simulink library "UAV_Control"  (R2018a)
settings: Solver=ode45  StartTime=0.0  StopTime=10.0  RelTol=1e-3  EnableMultiTasking=on
undefined symbols (not defined in the file or in its folder): alpha, dc_M_z, delta, Epsilon, g, Gamma, gamma_0, gamma_d_z, h, k, K, Ky, L, magnitude, mu1, mu2, nu, omega0, omega1, omega2, Phi0, Psi0, Rate, Rho_L, Rho_M, RPM_per, Sat, t0, t1, Tau, theta, theta0, Theta0, theta_0, theta_dot_M, theta_Max, theta_Min, Thrust_per, Tm, v, V0, X0, Xmax, Xmin, zeta1, zeta2, Zg
libraries: simulink x12, $bdroot x7
(part 1 of 2)
settings Model: Creator=ahmad  LastModifiedBy=Ahmad
settings DataIOCC: LimitDataPoints=on
settings OptimizationCC: LifeSpan=inf
settings DebuggingCC: AllowSymbolicDim=off  SFUnexpectedBacktrackingDiag=warning  SFNoUnconditionalDefaultTransitionDiag=warning  SFExecutionAtInitializationDiag=none
settings CodeAppCC: StateflowObjectComments=on
settings GRTTargetCC: TargetLangStandard=C89/C90 (ANSI)  GeneratePreprocessorConditionals=Disable all
settings ConfigComp: CovMetricSettings=dw  CovHtmlReporting=on  CovSaveCumulativeToWorkspaceVar=on  CovSaveSingleToWorkspaceVar=on  CovExternalEMLEnable=off

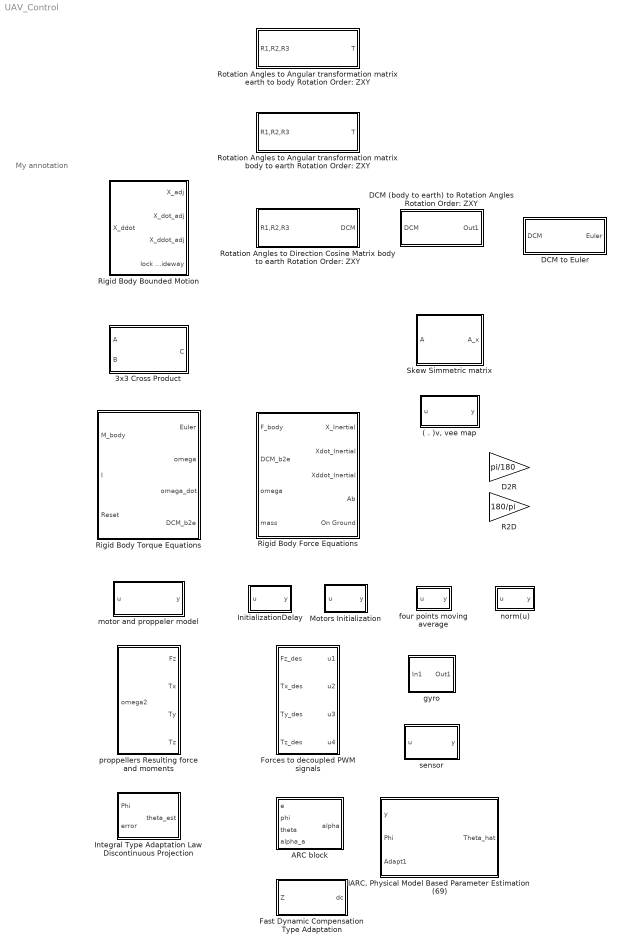
== system UAV_Control ==
  note: My annotation
  "( . )v, vee map" : Subsystem
  3x3 Cross Product : Subsystem  mask(3x3 Cross prduct){}
      mask Display:
      | port_label('input',1,'A','texmode','on')
      | port_label('input',2,'B','texmode','on')
      | port_label('output',1,'C','texmode','on')
  ARC block : Subsystem  mask(ARCBlock){k=k, theta_max=theta_Max, theta_min=theta_Min, epsilon=Epsilon, delta=delta}
      mask prompts: k "Linear Robuts gain:"; theta_max "Maximum parameters vector value:"; theta_min "Minimum parameters vector value:"; epsilon "Error bound Coefficient:"; delta "Uncertain Nonlinearities Bound:"
      mask help: Computes the ARC control part including: model compensation, stabalizing feedback, nonlinear robust feedback.
      mask Help:
      | h^2=(theta_max-theta_min)^2*phi^2+delta^2
      | alpha= alpha_a-( k + h^2/(4epsilon) )e/theta
      mask Display:
      | port_label('input',1,'e','texmode','on')
      | port_label('input',2,'\phi','texmode','on')
      | port_label('input',3,'\theta','texmode','on')
      | port_label('input',4,'\alpha_a','texmode','on')
      | port_label('output',1,'\alpha','texmode','on')
  "D2R " : Gain  Gain=pi/180  SaturateOnIntegerOverflow=on  OutDataTypeStr=Inherit: Same as input  ParamDataTypeStr=Inherit: Same as input
  DCM (body to earth) to Rotation Angles Rotation Order: ZXY : Subsystem  mask(DCM2Ang){}
      mask help: Get Euler angles from DCM in ZXY format.
      mask Help: Get Euler angles from DCM in ZXY format.
      mask Display:
      | port_label('input',1,'DCM_{be}','texmode','on')
      | port_label('output',1,'[R_1,R_2,R_3]','texmode','on')
  DCM to Euler : Subsystem
  Fast Dynamic Compensation Type Adaptation : Subsystem  mask{dc_M=dc_M_z, gamma_d=gamma_d_z}
      mask prompts: dc_M "Bound for the lumped model compensation errors"; gamma_d "Adaptation gain:"
      mask Help:
      | d ̂  ̇_c=Proj(γ_d z)=0             if      |d ̂_c |=d_cM  and d ̂_c z>0
      |                                 γ_d z      else
      | With γ_d>0 and |d ̂_c (0)|≤d_cM
      mask Display:
      | port_label('input',1,'e','texmode','on')
      | port_label('output',1,'d_c','texmode','on')
  Forces to decoupled PWM signals : Subsystem  mask(Forces2PWMSignals){K=K, Ky=Ky, L=L}
      mask prompts: K "Proppeler Force Coefficient:"; Ky "Proppeler Torque Coefficient:"; L "Arm Length:"
      mask help: Convertes the Quadcopter desired forces and moments to equivalent PWM signal.
      mask Help:
      | Convertes the Quadcopter desired forces and moments to equivalent PWM signal for a specific motors configuration.
      | 
      | Motors indices and rotation direction:
      | 1: back (CW)
      | 2: front (CW)
      | 3: left (CCW)
      | 4: righ (CCW)
      | 
      | parameters:
      | K: Proppeler Force Coefficient (N/(rad/s)^2)
      | Ky: Proppeler Torque Coefficient (N.m/(rad/s)^2)
      | L: Arm Length (m)
      | 
      | Inputs:
      | Fn=F/(4K)
      | Txn=Tx/(2LK)
      | Tyn=Ty/(2LK)
      | Tzn=Tz/(4Ky)
      | 
      | Outputs:
      | u1 =sqrt( Fn + Tyn + Tzn)
      | u2 = sqrt(Fn - Tyn + Tzn)
      | u3 = sqrt(Fn + Txn - Tzn)
      | u4 = sqrt(Fn - Txn - Tzn)
      | 
      | The PWM Duty cylce (ui) is limeted between 0 and 1.
      mask Display:
      | port_label('input',1,'F_{z,des}','texmode','on')
      | port_label('input',2,'\tau_{x,des}','texmode','on')
      | port_label('input',3,'\tau_{y,des}','texmode','on')
      | port_label('input',4,'\tau_{z,des}','texmode','on')
      | port_label('output',1,'u1','texmode','on')
      | port_label('output',2,'u2','texmode','on')
      | port_label('output',3,'u3','texmode','on')
      | port_label('output',4,'u4','texmode','on')
  "IARC, Physical Model Based Parameter Estimation (69)" : Subsystem  mask(Physical Model Based Parameter Estimation){mu1=mu1, mu2=mu2, alpha=alpha, nu=nu, gamma0=gamma_0, Rho_M=Rho_M, Rho_L=Rho_L, v=v, theta_0=theta_0, theta_max=theta_Max, theta_min=theta_Min, Theta_dot_M=theta_dot_M, Tau=Tau, t0=t0, Norm_ON=on}
      mask prompts: mu1 "forgetting factor, mu1:"; mu2 "RLS parameter, mu2:"; alpha "forgetting factor, alpha:"; nu "normalizing factor, nu:"; gamma0 "Initial adaptation gain:"; Rho_M "Upper bound for the adaptation gain:"; Rho_L "Lower bound for the adaptation gain:"; v "Eigenvector of Gamma_max:"; Theta_dot_M "Theta dot max:"; Tau "Filter time constant:"; t0 "Initialization Delay:"; Norm_ON "Use Normalized formula"
      mask Help:
      | Filtered system dynamics:
      | H_f (s)  is any stable LTI filter transfer function
      | x_f=H_f [x]
      | φ_f=H_f [φ(x)]
      | u_f=H_f [u]
      | 
      | y_p=x ̇_f−u_f
      | y ̂_p=φ_f^T θ ̂
      | Prediction error:
      | ϵ=y_p−y ̂_p
      | 
      | recursive estimation algorithms, the generalized parameter estimation algorithm (PAA) with covariance limiting:
      | 
      | θ ̂  ̇(t)=Γ(t) φ_f (t)ϵ(t)
      | D_Γ=μ_1 (t)Γ(t)−μ_2 (t)Γ(t) φ_f (t) φ_f (t)^T Γ(t)
      | Γ ̇(t)=D_Γ, if λ_M (Γ(t))<ρ_M  or v_M^T D_Γ v_M<0 )
      |          0        else
      | 
      | μ_1  and μ_2  are two non-negative functions
      | ρ_M  is a preset upper bound for the covariance matrix Γ(t)
      | μ_1  represents the forgetting factor (μ_1=0 for not forgetting)
      | μ_2: 1 stands for the standard least squares type estimation algorithm
      |        0 stands for  the gradient type estimation algorithm
      |        range: 0≤μ_2<2
      | Initialization of the covariance matrix: Γ(0)<ρ_M I_p
      | 
      | IARC designs completely separate the parameter estimation law design from the underlying robust control law to give better parameter estimates than possible with DARC designs. In addition, explicit on-line signal excitation level monitoring can be employed to significantly improve the accuracy of  parameter estimates.
      | 
      | Normalized Method:
      | θ ̂  ̇(t)=(Γ(t) φ_f (t)ϵ(t))/(1+νφ_f^T Γφ_f )
      | D_Γ=αΓ(t)−(Γ(t) φ_f (t) φ_f (t)^T Γ(t))/(1+νφ_f^T Γφ_f )
      | Γ ̇(t)=D_Γ, if λ_M (Γ(t))<ρ_M  or v_M^T D_Γ v_M<0
      |           0       else
      mask Display:
      | port_label('input',1,'y','texmode','on')
      | port_label('input',2,'\phi','texmode','on')
      | port_label('input',3,'Adapt','texmode','on')
      | 
      | port_label('output',1,'\theta_{hat}','texmode','on')
  InitializationDelay : Subsystem  mask(InitializationDelay){t0=t0}
      mask prompts: t0 "Initialization delay:"
      mask help: Applays a delay before passing the first signal.
      mask Help: Applays a delay (t0) before passing the first signal
      mask Display:
      | port_label('input',1,'u','texmode','on')
      | port_label('output',1,'y','texmode','on')
  Integral Type Adaptation Law Discontinuous Projection : Subsystem  mask(IntegralTypeAdaptationLaw){theta=theta, theta0=theta0, theta_max=theta_Max, theta_min=theta_Min, gamma=Gamma, t0=t0, Adaptation_ON=on}
      mask prompts: theta "Actual value of theta:"; theta0 "Initial value of theta:"; theta_max "Maximum value of theta:"; theta_min "Minimum value of theta:"; gamma "Adaptation Rate:"; t0 "Initialization Delay:"; Adaptation_ON "Activate adaptation:"
      mask help: Applies an Integral-type adaptation law with discontinuous projection on the parameter theta.
      mask Help:
      | Applies an Integral-type adaptation law with discontinuous projection on the parameter theta.
      | 
      | theta_est_dot=Gamma*Phi*e
      | theta=proj( int(theta_estdot) )
      | 
      | theta_min < theta_est <  theta_max
      | 
      | Parameters:
      | 
      | Gamma: nxn diagonal matrix, adaptaion rate.
      | theta_min: nx1 vector, minimum value of the estimated vector.
      | theta_max: nx1 vector, maximum value of the estimated vector.
      | theta0: nx1 vector, initial value of the estimated vector.
      | theta: nx1 vector, actual value of the estimated vector.
      | Adaptation_On: controls the use of the adaptation law (1: active, 0: inactive)
      | 
      | Inputs:
      | Phi: regressor vector, theta0, nx1.
      | e: state error, scalar.
      | 
      | Outputs:
      | theta_est: estimated value of the parameters vector.
      mask Display:
      | port_label('input',1,'\phi','texmode','on')
      | port_label('input',2,'e','texmode','on')
      | port_label('output',1,'\theta_{hat}','texmode','on')
  "Motors Initialization " : Subsystem  mask(MotorsInitialization){t0=t0, t1=t1, Sat=Sat, Parameter4=Rate}
      mask prompts: t0 "Initialization delay:"; t1 "Input pass time:"; Sat "Signal saturation during initialization:"; Parameter4 "Signal rate during initialization:"
      mask help: Delays the pass out of the input while passing a warmup rizing signal.
      mask Display:
      | port_label('input',1,'u','texmode','on')
      | port_label('output',1,'y','texmode','on')
  "R2D " : Gain  Gain=180/pi  SaturateOnIntegerOverflow=on  OutDataTypeStr=Inherit: Same as input  ParamDataTypeStr=Inherit: Same as input
  Rigid Body Force Equations : Subsystem  mask(Rigid body force equations){g=g, h0=Zg, X0=X0, X_min=Xmin, X_max=Xmax, V0=V0}
      mask prompts: g "Gravity:"; h0 "Ground height:"; X0 "Initial Position:"; X_min "Position Lower Bound:"; X_max "Position Upper Bound:"; V0 "Initial Velocity:"
      mask help: Determines the translational motion of a 6DOF rigid body.
      mask Help:
      | a_b= Fb/m-omega x V_b
      | 
      | 
      | 
      | Fb=R_eb*[0 0 -mg]+[0 0 Fz]+R_eb*Fd_e
      | 
      | where Fz is the thrust force (in body z direction)
      | and Fd_e is a force disturbace in the earth frame.
      | 
      | a_e = R_be*a_b
      mask Display:
      | port_label('input',1,'F_b (N)','texmode','on')
      | port_label('input',2,'DCM_{b2e}','texmode','on')
      | port_label('input',3,'\omega (rad/s)','texmode','on')
      | port_label('input',4,'m (kg)','texmode','on')
      | 
      | port_label('output',1,'X_e (m)','texmode','on')
      | port_label('output',2,'V_e (m/s)','texmode','on')
      | port_label('output',3,'a_e (m/s^2)','texmode','on')
      | port_label('output',4,'a_b (m/s^2)','texmode','on')
      | port_label('output',5,'On Ground','texmode','on')
  "Rigid Body Torque Equations " : Subsystem  mask(Rotational motion of rigid body){Euler0=[Phi0 Theta0 Psi0], omega0=omega0}
      mask prompts: Euler0 "Initial euler angles:"; omega0 "Initial angular velocites:"
      mask help: Determines the rotational motion of a 6DOF rigid body.
      mask Help:
      | alpha=Mb/I - omega x omega
      | omega=alpha_dot
      | Euler=omega_dot
      mask Display:
      | port_label('input',1,'M_b (N.m)','texmode','on')
      | port_label('input',2,'I (kg/m^2)','texmode','on')
      | port_label('input',3,'Reset','texmode','on')
      | 
      | port_label('output',1,'\phi,\theta,\psi (rad)','texmode','on')
      | port_label('output',2,'\omega (rad/s)','texmode','on')
      | port_label('output',3,'\alpha (rad/s^2)','texmode','on')
      | port_label('output',4,'DCM_{b2e}','texmode','on')
  Rigid Body Bounded Motion : Subsystem  mask{Parameter1=Zg, Parameter2=X0, Parameter3=V0, Parameter4=Xmin, Parameter5=Xmax}
      mask prompts: Parameter1 "Ground level:"; Parameter2 "Initial Possition:"; Parameter3 "Initial Velocity:"; Parameter4 "Position Lower Bound:"; Parameter5 "Position Upper Bound:"
      mask help: Bounds the motion of a rigid body in space: [Xmin Xmax]
      mask Help:
      | Bounds the motion of a rigid body in space.
      | 
      | Dialog box parameters:
      | Zg: A scalar value for ground height (m).
      | X0 (x,y,z): tree-element vector, initial position of the body (m).
      | V0(vx,vy,vz): tree-element vector, for the initial velocity of the body (m/s).
      | Xmin: tree-element vector for the position lower bound (m).
      | Xmax: tree-element vector for the position upper bound (m).
      | 
      | Input:
      | First: Contains the acceleration of the body resolved into the earth coordinate frame, (A, m/s).
      | 
      | Outputs:
      | First: Contains the bounded position of the body resolved into the earth coordinate frame, tree-element vector, (X, m).
      | Second: Contains the bounded velocitiy of the body resolved into the earth coordinate frame, tree-element vector, (Vadj, m/s).
      | Third: Contains the bounded acceleration of the body resolved into the earth coordinate frame, tree-element vector, (Aadj, m/s2).
      mask Display:
      | port_label('input',1,'A','texmode','on');
      | port_label('output',1,'X_{b}','texmode','on');
      | port_label('output',2,'V_{adj}','texmode','on');
      | port_label('output',3,'A_{adj}','texmode','on');
      | port_label('output',4,'On ground','texmode','on');
  Rotation Angles to Angular transformation matrix body to earth Rotation Order: ZXY : Subsystem  mask(Ang2T){}
      mask help: Determine the 3-by-3 Angular transformation matrix (T) from a given set of rotation angles (ZXY).
      mask Help:
      | Generate the Angular Transformation matrix (T) from the Euler angles. Order of transformation. body to earth.
      | ZYX
      | 
      | T_B2E = [         cos(theta)             0          -sin(theta)
      |                  -sin(theta)*tan(phi)      1    -cos(theta)*tan(phi)
      |                    sin(theta)/cos(phi)     0     cos(theta)/cos(phi) ]
      mask Display:
      | port_label('input',1,'[R_1,R_2,R_3]','texmode','on')
      | port_label('output',1,'T_{eb}','texmode','on')
  Rotation Angles to Angular transformation matrix earth to body Rotation Order: ZXY : Subsystem  mask(Ang2T){}
      mask help: Determine the 3-by-3 Angular transformation matrix (T) from a given set of rotation angles (ZXY).
      mask Help:
      | Generate the Angular transformation matrix  (T) from the Euler angles. Order of transformation.
      | ZXY
      | 
      | T_B2E = [         cos(theta)             0          -sin(theta)*cos(phi)
      |                                0                       1                    sin(phi)
      |                          sin(theta)              0            cos(theta)*cos(phi) ]
      mask Display:
      | port_label('input',1,'[R_1,R_2,R_3]','texmode','on')
      | port_label('output',1,'T_{eb}','texmode','on')
  Rotation Angles to Direction Cosine Matrix body to earth Rotation Order: ZXY : Subsystem  mask(Ang2DCM){}
      mask help: Determine the 3-by-3 direction cosine matrix (DCM) from a given set of rotation angles.
      mask Help:
      | Generate the Direction Cosine Matrix (DCM) from the Euler angles. Order of transformation: ZXY.
      | ZYX >> phi theta psi
      | 
      | DCM_B2E=[cos(theta)cos(psi), sin(phi)sin(theta)cos(psi)-cos(phi)sin(psi), cos(phi)sin(theta)cos(psi)+sin(phi)sin(psi)
      |                       cos(theta)sin(psi), sin(phi)sin(theta)sin(psi)+cos(phi)cos(psi), cos(phi)sin(theta)sin(psi)-sin(phi)cos(psi)
      |                             -sin(theta)      ,                 sin(phi)cos(theta)                          ,                           cos(phi)cos(theta)               ]
      | 'texmode','on'
      mask Display:
      | port_label('input',1,'[R_1,R_2,R_3]','texmode','on')
      | port_label('output',1,'DCM_{eb}','texmode','on')
  Skew Simmetric matrix : Subsystem
  four points moving average : Subsystem
  gyro : Subsystem
  motor and proppeler model : Subsystem  mask{CorrMode=off, Thrust=Thrust_per, RPM=RPM_per, TimeConstant=Tm}
      mask prompts: CorrMode "Correction mode"; Thrust "Thrust percentage data:"; RPM "RPM percentage data:"; TimeConstant "Motor time constant:"
      mask init:
      | if CorrMode
      |     c=1;
      | else
      |     c=0;
      | end
      mask Display:
      | port_label('input',1,'Duty cycle','texmode','on')
      | port_label('output',1,'\omega^2','texmode','on')
  norm(u) : Subsystem
  proppellers Resulting force and moments : Subsystem  mask(QuadcopterMotorsResultingForces&Moments){K=K, Ky=Ky, L=L}
      mask prompts: K "Proppeler Force Coefficient:"; Ky "Proppeler Torque Coefficient:"; L "Arm Length:"
      mask help: Calculates the resulting forces & moments of the quadcopter motors.
      mask Help:
      | Calculates the resulting forces & moments of the quadcopter motors given the motors speed.
      | 
      | parameters:
      | K: Proppeler Force Coefficient (N/(rad/s)^2)
      | Ky: Proppeler Torque Coefficient (N.m/(rad/s)^2)
      | L: Arm Length (m)
      | 
      | Fz=K*(omega1^2+omega2^2+omega3^2+omega4^2)
      | Tx=K*L*(omega3^2-omega4^2)
      | Ty=K*L*(omega1^2-omega2^2)
      | Tz=Ky*(omega1^2+omega2^2-omega3^2-omega4^2)
      | 
      | Input:
      | omega^2: a four elements vector contaning the squared velocity of each of the four motors.
      | 
      | Outputs:
      | all the outputs are in body frame.
      | Fz: Total force in the Z direction.
      | Tx: Moment about the body X-axis.
      | Ty: Moment about the body Y-axis.
      | Tz: Moment about the body Z-axis.
      mask Display:
      | port_label('input',1,'\omega^2','texmode','on')
      | port_label('output',1,'F_z','texmode','on')
      | port_label('output',2,'\tau_x','texmode','on')
      | port_label('output',3,'\tau_y','texmode','on')
      | port_label('output',4,'\tau_z','texmode','on')
  sensor : Subsystem

== system UAV_Control/( . )v, vee map ==
  u : Inport
  12 (D_psi) : Selector  NumberOfDimensions=2  InputPortWidth=3  IndexOptions=Index vector (dialog),Index vector (dialog)  Indices=1,2  OutputSizes=1,1
  23 (D_phi) : Selector  NumberOfDimensions=2  InputPortWidth=3  IndexOptions=Index vector (dialog),Index vector (dialog)  Indices=2,3  OutputSizes=1,1
  31 (D_theta) : Selector  NumberOfDimensions=2  InputPortWidth=3  IndexOptions=Index vector (dialog),Index vector (dialog)  Indices=3,1  OutputSizes=1,1
  Mux : Mux  Inputs=3
  y : Outport
  wires:
  12 (D_psi)/1 -> Mux/3
  31 (D_theta)/1 -> Mux/2
  23 (D_phi)/1 -> Mux/1
  u/1 -> 31 (D_theta)/1, 23 (D_phi)/1, 12 (D_psi)/1
  Mux/1 -> y/1

== system UAV_Control/3x3 Cross Product ==
  A : Inport
  B : Inport  Port=2
  "A " : InportShadow
  "B " : InportShadow  Port=2
  Subsystem : Subsystem
  Subsystem1 : Subsystem
  Sum : Sum  Inputs=+|-  SaturateOnIntegerOverflow=on  InputSameDT=on  OutDataTypeStr=Inherit: Same as first input
  C : Outport
  wires:
  Subsystem1/1(Out1) -> Sum/2
  Subsystem/1(Out1) -> Sum/1
  A/1 -> Subsystem/1(A)
  B/1 -> Subsystem/2(B)
  Sum/1 -> C/1
  "A "/1 -> Subsystem1/1(A)
  "B "/1 -> Subsystem1/2(B)

== system UAV_Control/ARC block ==
  e : Inport
  phi : Inport  Port=2
  theta : Inport  Port=3
  alpha_a : Inport  Port=4
  1 : Scope
  Add : Sum  Inputs=--+
  Mux1 : Mux
  alpha_S1 : Gain  Gain=k
  e/theta : Product  Inputs=*/
  h^2 : Subsystem
      mask Display:
      | port_label('input',1,'e/\theta','texmode','on')
      | port_label('input',2,'\phi','texmode','on')
      | 
      | port_label('output',1,'\alpha_{s2}','texmode','on')
  alpha : Outport
  wires:
  e/theta/1 -> alpha_S1/1, h^2/1(e)
  alpha_a/1 -> Mux1/3, Add/3
  Mux1/1 -> 1/1
  Add/1 -> Mux1/4, alpha/1
  alpha_S1/1 -> Mux1/1, Add/1
  h^2/1("alpha_s2 ") -> Mux1/2, Add/2
  e/1 -> e/theta/1
  theta/1 -> e/theta/2
  phi/1 -> h^2/2(phi)

== system UAV_Control/DCM (body to earth) to Rotation Angles Rotation Order: ZXY ==
  DCM : Inport  Unit=1
  "AxisRotDefault " : Subsystem  TreatAsAtomicUnit=on
  "AxisRotZeroR3 " : Subsystem  TreatAsAtomicUnit=on
  "Get DCM Values " : Subsystem
  If : If  IfExpression=(u1>=1)|(u1<=-1)
  Merge : Merge
  Selector4 : Selector  InputPortWidth=7  IndexOptions=Index vector (dialog)  Indices=3  OutputSizes=1
  Out1 : Outport  Unit=rad
  wires:
  "AxisRotZeroR3 "/1(Out1) -> Merge/1
  "AxisRotDefault "/1(Out1) -> Merge/2
  If/2 -> "AxisRotDefault "/Action
  Merge/1 -> Out1/1
  Selector4/1 -> If/1  "r21"
  "Get DCM Values "/1(Out1) -> "AxisRotZeroR3 "/1(In1), "AxisRotDefault "/1(In1), Selector4/1
  DCM/1 -> "Get DCM Values "/1(In1)
  If/1 -> "AxisRotZeroR3 "/Action

== system UAV_Control/DCM to Euler ==
  DCM : Inport
  12 : Selector  NumberOfDimensions=2  InputPortWidth=3  IndexOptions=Index vector (dialog),Index vector (dialog)  Indices=1,2  OutputSizes=1,1
  22 : Selector  NumberOfDimensions=2  InputPortWidth=3  IndexOptions=Index vector (dialog),Index vector (dialog)  Indices=2,2  OutputSizes=1,1
  31 : Selector  NumberOfDimensions=2  InputPortWidth=3  IndexOptions=Index vector (dialog),Index vector (dialog)  Indices=3,1  OutputSizes=1,1
  32 : Selector  NumberOfDimensions=2  InputPortWidth=3  IndexOptions=Index vector (dialog),Index vector (dialog)  Indices=3,2  OutputSizes=1,1
  33 : Selector  NumberOfDimensions=2  InputPortWidth=3  IndexOptions=Index vector (dialog),Index vector (dialog)  Indices=3,3  OutputSizes=1,1
  Mux : Mux  Inputs=3
  Mux1 : Mux  Inputs=3
  Mux2 : Mux  Inputs=3
  phi : Fcn  Expr=asin(u(1))
  psi : Fcn  Expr=atan2(-u(1)/cos(u(3)),u(2)/cos(u(3)))
  theta : Fcn  Expr=atan2(-u(1)/cos(u(3)),u(2)/cos(u(3)))
  Euler : Outport
  wires:
  psi/1 -> Mux2/3
  Mux1/1 -> psi/1
  Mux/1 -> theta/1
  33/1 -> Mux/2
  32/1 -> phi/1
  DCM/1 -> 12/1, 22/1, 33/1, 32/1, 31/1
  22/1 -> Mux1/2
  12/1 -> Mux1/1
  phi/1 -> Mux1/3, Mux2/1, Mux/3
  theta/1 -> Mux2/2
  31/1 -> Mux/1
  Mux2/1 -> Euler/1

== system UAV_Control/Fast Dynamic Compensation Type Adaptation ==
  Z : Inport
  Gain : Gain  Gain=gamma_d
  Integrator : Integrator  LimitOutput=on  UpperSaturationLimit=dc_M  LowerSaturationLimit=-dc_M
  dc : Outport
  wires:
  Integrator/1 -> dc/1
  Z/1 -> Gain/1
  Gain/1 -> Integrator/1

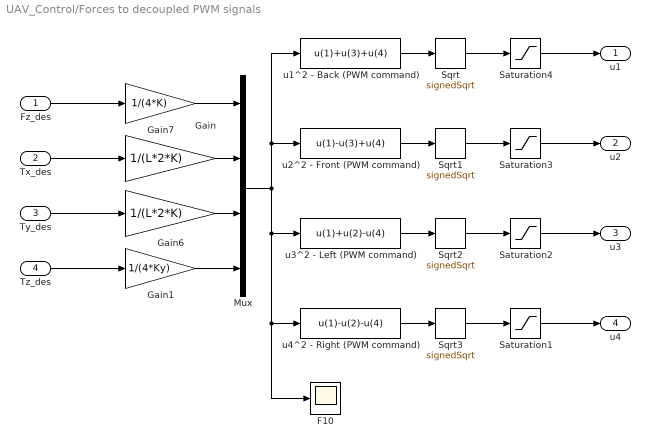
== system UAV_Control/Forces to decoupled PWM signals ==
  Fz_des : Inport
  Tx_des : Inport  Port=2
  Ty_des : Inport  Port=3
  Tz_des : Inport  Port=4
  F10 : Scope
  Gain : Gain  Gain=1/(L*2*K)
  Gain1 : Gain  Gain=1/(4*Ky)
  Gain6 : Gain  Gain=1/(L*2*K)
  Gain7 : Gain  Gain=1/(4*K)
  Mux : Mux
  Saturation{1..4} (4 alike) : Saturate  UpperLimit=1  LowerLimit=0
  Sqrt{,1..3} (4 alike) : Sqrt  Operator=signedSqrt  OutputSignalType=real  SaturateOnIntegerOverflow=on
  u1^2 - Back (PWM command) : Fcn  Expr=u(1)+u(3)+u(4)
  u2^2 - Front (PWM command) : Fcn  Expr=u(1)-u(3)+u(4)
  u3^2 - Left (PWM command) : Fcn  Expr=u(1)+u(2)-u(4)
  u4^2 - Right (PWM command) : Fcn  Expr=u(1)-u(2)-u(4)
  u1 : Outport
  u2 : Outport  Port=2
  u3 : Outport  Port=3
  u4 : Outport  Port=4
  wires:
  Sqrt1/1 -> Saturation3/1
  Sqrt2/1 -> Saturation2/1
  Sqrt3/1 -> Saturation1/1
  Sqrt/1 -> Saturation4/1
  u4^2 - Right (PWM command)/1 -> Sqrt3/1
  u3^2 - Left (PWM command)/1 -> Sqrt2/1
  u2^2 - Front (PWM command)/1 -> Sqrt1/1
  u1^2 - Back (PWM command)/1 -> Sqrt/1
  Saturation1/1 -> u4/1
  Saturation3/1 -> u2/1
  Saturation2/1 -> u3/1
  Saturation4/1 -> u1/1
  Gain7/1 -> Mux/1
  Gain1/1 -> Mux/4
  Gain6/1 -> Mux/3
  Gain/1 -> Mux/2
  Mux/1 -> u1^2 - Back (PWM command)/1, u2^2 - Front (PWM command)/1, u3^2 - Left (PWM command)/1, u4^2 - Right (PWM command)/1, F10/1
  Tz_des/1 -> Gain1/1
  Ty_des/1 -> Gain6/1
  Fz_des/1 -> Gain7/1
  Tx_des/1 -> Gain/1

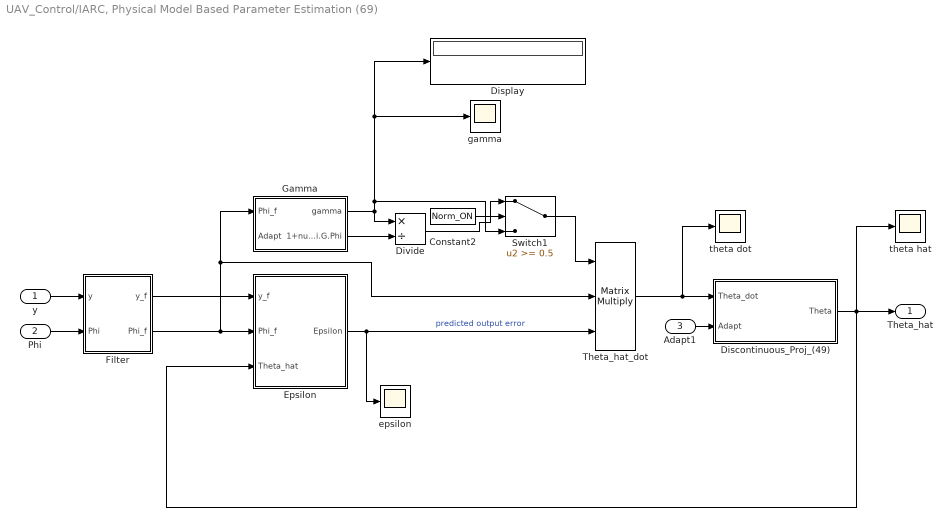
== system UAV_Control/IARC, Physical Model Based Parameter Estimation (69) ==
  y : Inport
  Phi : Inport  Port=2
  Adapt1 : Inport  Port=3
  Constant2 : Constant  Value=Norm_ON
  Discontinuous_Proj_(49) : Subsystem
  Display : Display
  Divide : Product  Inputs=*/
  Epsilon : Subsystem
  Filter : Subsystem
  Gamma : Subsystem
  Switch1 : Switch  Threshold=0.5
  Theta_hat_dot : Product  Inputs=3  Multiplication=Matrix(*)
  "epsilon  " : Scope
  gamma : Scope
  theta dot : Scope
  theta hat : Scope
  Theta_hat : Outport
  wires:
  Gamma/2(" 1+nu.Phi.G.Phi") -> Divide/2
  Divide/1 -> Switch1/1
  Switch1/1 -> Theta_hat_dot/1
  Gamma/1(" gamma") -> Divide/1, Switch1/3, gamma/1, Display/1
  Constant2/1 -> Switch1/2
  Theta_hat_dot/1 -> theta dot/1, Discontinuous_Proj_(49)/1(Theta_dot)
  y/1 -> Filter/1(y)
  Phi/1 -> Filter/2("Phi ")
  Filter/1(y_f) -> Epsilon/1(y_f)
  Discontinuous_Proj_(49)/1(Theta) -> theta hat/1, Theta_hat/1, Epsilon/3(Theta_hat)
  Epsilon/1(Epsilon) -> Theta_hat_dot/3, "epsilon  "/1  "predicted output error"
  Filter/2(Phi_f) -> Theta_hat_dot/2, Gamma/1(Phi_f), Epsilon/2(Phi_f)
  Adapt1/1 -> Discontinuous_Proj_(49)/2(Adapt)

== system UAV_Control/InitializationDelay ==
  u : Inport
  Clock : Clock
  Compare To Constant2 : simulink/Logic and Bit Operations/Compare To Constant  relop=>=  const=t0  OutDataTypeStr=boolean
  Data Type Conversion : DataTypeConversion
  Product : Product
  y : Outport
  wires:
  Product/1 -> y/1
  Data Type Conversion/1 -> Product/2
  Clock/1 -> Compare To Constant2/1
  Compare To Constant2/1 -> Data Type Conversion/1
  u/1 -> Product/1

== system UAV_Control/Integral Type Adaptation Law Discontinuous Projection ==
  Phi : Inport
  error : Inport  Port=2
  Constant : Constant  Value=gamma
  Constant2 : Constant  Value=Adaptation_ON
  Discontinuous Projection : Integrator  InitialCondition=theta0  LimitOutput=on  UpperSaturationLimit=theta_max  LowerSaturationLimit=theta_min
  InitializationDelay : $bdroot/InitializationDelay  t0=t0
  Product1 : Product  Inputs=3  Multiplication=Matrix(*)
  Switch1 : Switch  Criteria=u2 ~= 0
  real : Constant  Value=theta
  theta_est : Outport
  wires:
  Switch1/1 -> theta_est/1
  Discontinuous Projection/1 -> Switch1/1
  Phi/1 -> Product1/2
  Product1/1 -> InitializationDelay/1
  InitializationDelay/1 -> Discontinuous Projection/1
  Constant2/1 -> Switch1/2
  real/1 -> Switch1/3
  error/1 -> Product1/3
  Constant/1 -> Product1/1

== system UAV_Control/Motors Initialization  ==
  u : Inport
  Clock : Clock
  Compare To Constant1 : simulink/Logic and Bit Operations/Compare To Constant  relop=<=  const=t1  OutDataTypeStr=boolean
  Compare To Constant2 : simulink/Logic and Bit Operations/Compare To Constant  relop=>=  const=t0  OutDataTypeStr=boolean
  Constant : Constant  Value=0
  Gain : Gain  Gain=Rate
  Saturation : Saturate  UpperLimit=Sat  LowerLimit=0
  Scope : Scope
  Scope1 : Scope
  Switch : Switch  Criteria=u2 > Threshold  Threshold=0.5
  Switch1 : Switch  Criteria=u2 > Threshold  Threshold=0.5
  y : Outport
  wires:
  u/1 -> Switch1/3
  Clock/1 -> Compare To Constant1/1, Compare To Constant2/1, Gain/1
  Compare To Constant2/1 -> Switch/2
  Gain/1 -> Saturation/1
  Saturation/1 -> Switch/1
  Constant/1 -> Switch/3
  Compare To Constant1/1 -> Switch1/2
  Switch1/1 -> Scope1/1, y/1
  Switch/1 -> Switch1/1, Scope/1

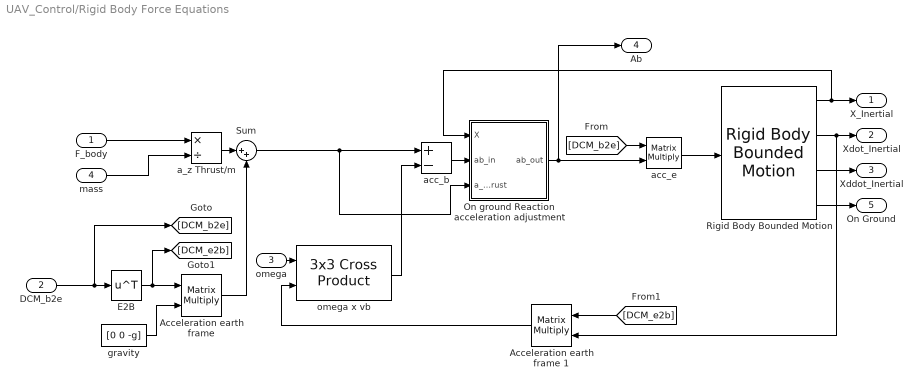
== system UAV_Control/Rigid Body Force Equations ==
  F_body : Inport
  DCM_b2e : Inport  Port=2
  omega : Inport  Port=3
  mass : Inport  Port=4
  Acceleration earth frame : Product  Multiplication=Matrix(*)
  Acceleration earth frame 1 : Product  Multiplication=Matrix(*)
  E2B : Math  Operator=transpose  SaturateOnIntegerOverflow=on
  On ground Reaction acceleration adjustment : Subsystem
  Rigid Body Bounded Motion : $bdroot/Rigid Body Bounded Motion  Parameter1=Zg  Parameter2=X0  Parameter3=V0  Parameter4=Xmin  Parameter5=Xmax
  Sum : Sum  Inputs=|++
  a_z Thrust/m : Product  Inputs=*/
  acc_b : Sum  Inputs=+-
  acc_e : Product  Multiplication=Matrix(*)
  gravity : Constant  Value=[0 0 -g]
  omega x vb : $bdroot/3x3 Cross Product
  X_Inertial : Outport
  Xdot_Inertial : Outport  Port=2
  Xddot_Inertial : Outport  Port=3
  Ab : Outport  Port=4
  On Ground : Outport  Port=5
  wires:
  acc_e/1 -> Rigid Body Bounded Motion/1
  omega x vb/1 -> acc_b/2
  Acceleration earth frame 1/1 -> omega x vb/2
  Rigid Body Bounded Motion/2 -> Xdot_Inertial/1, Acceleration earth frame 1/2
  [DCM_e2b] -> Acceleration earth frame 1/1
  a_z Thrust/m/1 -> Sum/1
  [DCM_b2e] -> acc_e/1
  On ground Reaction acceleration adjustment/1(ab_out) -> Ab/1, acc_e/2
  omega/1 -> omega x vb/1
  acc_b/1 -> On ground Reaction acceleration adjustment/2(ab_in)
  E2B/1 -> Acceleration earth frame/1, [DCM_e2b]
  F_body/1 -> a_z Thrust/m/1
  gravity/1 -> Acceleration earth frame/2
  Acceleration earth frame/1 -> Sum/2
  DCM_b2e/1 -> E2B/1, [DCM_b2e]
  Sum/1 -> acc_b/1, On ground Reaction acceleration adjustment/3(a_thrust)
  Rigid Body Bounded Motion/1 -> On ground Reaction acceleration adjustment/1(X), X_Inertial/1
  Rigid Body Bounded Motion/3 -> Xddot_Inertial/1
  mass/1 -> a_z Thrust/m/2
  Rigid Body Bounded Motion/4 -> On Ground/1

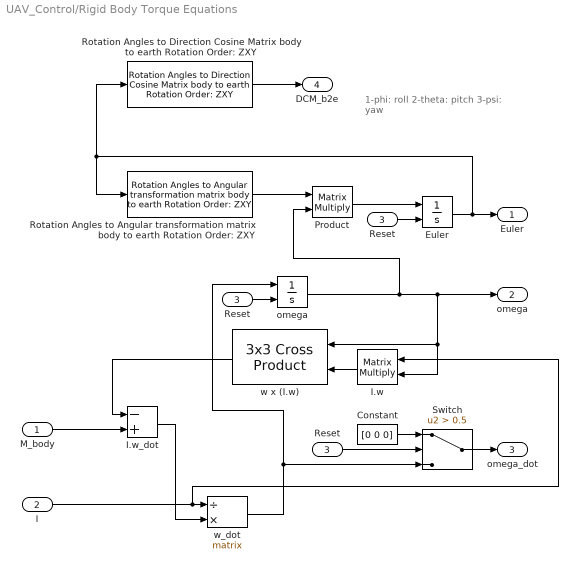
== system UAV_Control/Rigid Body Torque Equations  ==
  note: 1-phi: roll
      | 2-theta: pitch
      | 3-psi: yaw
  M_body : Inport
  I : Inport  Port=2
  Reset : Inport  Port=3
  Constant : Constant  Value=[0 0 0]
  Euler : Integrator  ExternalReset=level hold  InitialCondition=[Phi0 Theta0 Psi0]  UpperSaturationLimit=2  LowerSaturationLimit=-2
  I.w : Product  Multiplication=Matrix(*)
  I.w_dot : Sum  Inputs=-+
  Product : Product  Multiplication=Matrix(*)
  "Reset " : InportShadow  Port=3
  "Reset  " : InportShadow  Port=3
  Rotation Angles to Angular transformation matrix body to earth Rotation Order: ZXY : $bdroot/Rotation Angles to Angular transformation matrix body to earth Rotation Order: ZXY
  Rotation Angles to Direction Cosine Matrix body to earth Rotation Order: ZXY : $bdroot/Rotation Angles to Direction Cosine Matrix body to earth Rotation Order: ZXY
  Switch : Switch  Criteria=u2 > Threshold  Threshold=0.5
  "omega  " : Integrator  ExternalReset=level hold  InitialCondition=omega0  UpperSaturationLimit=2  LowerSaturationLimit=-2
  w x (I.w) : $bdroot/3x3 Cross Product
  w_dot : Product  Inputs=/*  Multiplication=Matrix(*)
  "Euler " : Outport
  omega : Outport  Port=2
  omega_dot : Outport  Port=3
  DCM_b2e : Outport  Port=4
  wires:
  w x (I.w)/1 -> I.w_dot/1
  M_body/1 -> I.w_dot/2
  Euler/1 -> "Euler "/1, Rotation Angles to Direction Cosine Matrix body to earth Rotation Order: ZXY/1, Rotation Angles to Angular transformation matrix body to earth Rotation Order: ZXY/1
  Rotation Angles to Angular transformation matrix body to earth Rotation Order: ZXY/1 -> Product/1
  w_dot/1 -> "omega  "/1, Switch/3
  Product/1 -> Euler/1
  I/1 -> I.w/1, w_dot/1
  "omega  "/1 -> Product/2, I.w/2, w x (I.w)/1, omega/1
  Constant/1 -> Switch/1
  Reset/1 -> Switch/2
  Switch/1 -> omega_dot/1
  "Reset "/1 -> "omega  "/2
  "Reset  "/1 -> Euler/2
  Rotation Angles to Direction Cosine Matrix body to earth Rotation Order: ZXY/1 -> DCM_b2e/1
  I.w/1 -> w x (I.w)/2
  I.w_dot/1 -> w_dot/2

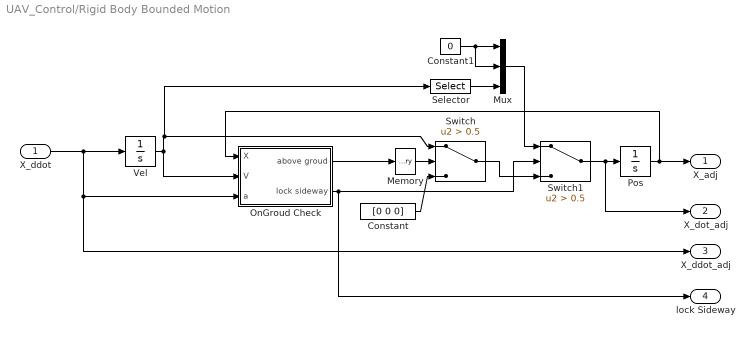
== system UAV_Control/Rigid Body Bounded Motion ==
  X_ddot : Inport
  Constant : Constant  Value=[0 0 0]
  Constant1 : Constant  Value=0
  Memory : Memory
  Mux : Mux  Inputs=3
  OnGroud Check : Subsystem
  Pos : Integrator  InitialCondition=X0  LimitOutput=on  UpperSaturationLimit=Xmax  LowerSaturationLimit=Xmin
  Selector : Selector  InputPortWidth=3  IndexOptions=Index vector (dialog)  Indices=3  OutputSizes=1
  Switch : Switch  Criteria=u2 > Threshold  Threshold=0.5
  Switch1 : Switch  Criteria=u2 > Threshold  Threshold=0.5
  Vel : Integrator  InitialCondition=V0
  X_adj : Outport
  X_dot_adj : Outport  Port=2
  X_ddot_adj : Outport  Port=3
  lock Sideway : Outport  Port=4
  wires:
  Memory/1 -> Switch/2
  OnGroud Check/1(above groud) -> Memory/1
  Switch1/1 -> X_dot_adj/1, Pos/1
  Vel/1 -> OnGroud Check/2(V), Selector/1, Switch/1
  X_ddot/1 -> X_ddot_adj/1, OnGroud Check/3(a), Vel/1
  Pos/1 -> OnGroud Check/1(X), X_adj/1
  Constant/1 -> Switch/3
  OnGroud Check/2(lock sideway) -> lock Sideway/1, Switch1/2
  Switch/1 -> Switch1/3
  Mux/1 -> Switch1/1
  Constant1/1 -> Mux/2, Mux/1
  Selector/1 -> Mux/3

== system UAV_Control/Rotation Angles to Angular transformation matrix body to earth Rotation Order: ZXY ==
  R1,R2,R3 : Inport  PortDimensions=3
  Fcn1 : Fcn  Expr=0
  Fcn11 : Fcn  Expr=u(5)
  Fcn13 : Fcn  Expr=-u(2)
  Fcn21 : Fcn  Expr=-u(2)*u(1)/u(4)
  Fcn22 : Fcn  Expr=1
  Fcn23 : Fcn  Expr=-u(5)*u(1)/u(4)
  Fcn3 : Fcn  Expr=u(5)/u(4)
  Fcn32 : Fcn  Expr=0
  Fcn33 : Fcn  Expr=u(2)/u(4)
  Mux : Mux  Inputs=2
  Subsystem : Subsystem
  sincos : Trigonometry  Operator=sincos
  T : Outport  PortDimensions=[3,3]
  wires:
  Fcn3/1 -> Subsystem/9(In9)
  Fcn23/1 -> Subsystem/8(In8)
  Fcn1/1 -> Subsystem/6(In6)
  Fcn22/1 -> Subsystem/5(In5)
  Fcn13/1 -> Subsystem/7(In7)
  Fcn32/1 -> Subsystem/4(In4)
  Fcn33/1 -> Subsystem/3(In3)
  Fcn21/1 -> Subsystem/2(In2)
  Fcn11/1 -> Subsystem/1(In1)
  Mux/1 -> Fcn1/1, Fcn3/1, Fcn23/1, Fcn13/1, Fcn32/1, Fcn11/1, Fcn21/1, Fcn33/1, Fcn22/1
  sincos/2 -> Mux/2
  sincos/1 -> Mux/1
  Subsystem/1(Out1) -> T/1
  R1,R2,R3/1 -> sincos/1

== system UAV_Control/Rotation Angles to Angular transformation matrix earth to body Rotation Order: ZXY ==
  R1,R2,R3 : Inport  PortDimensions=3
  Fcn1 : Fcn  Expr=0
  Fcn11 : Fcn  Expr=u(5)
  Fcn12 : Fcn  Expr=0
  Fcn13 : Fcn  Expr=u(2)
  Fcn2 : Fcn  Expr=u(1)
  Fcn22 : Fcn  Expr=1
  Fcn3 : Fcn  Expr=u(4)*u(5)
  Fcn31 : Fcn  Expr=-u(2)*u(4)
  Fcn32 : Fcn  Expr=0
  Mux : Mux  Inputs=2
  Subsystem : Subsystem
  sincos : Trigonometry  Operator=sincos
  T : Outport  PortDimensions=[3,3]
  wires:
  R1,R2,R3/1 -> sincos/1
  Subsystem/1(Out1) -> T/1
  sincos/1 -> Mux/1
  sincos/2 -> Mux/2
  Mux/1 -> Fcn22/1, Fcn13/1, Fcn11/1, Fcn12/1, Fcn32/1, Fcn2/1, Fcn3/1, Fcn31/1, Fcn1/1
  Fcn11/1 -> Subsystem/1(In1)
  Fcn12/1 -> Subsystem/2(In2)
  Fcn13/1 -> Subsystem/3(In3)
  Fcn32/1 -> Subsystem/4(In4)
  Fcn31/1 -> Subsystem/7(In7)
  Fcn22/1 -> Subsystem/5(In5)
  Fcn1/1 -> Subsystem/6(In6)
  Fcn2/1 -> Subsystem/8(In8)
  Fcn3/1 -> Subsystem/9(In9)

== system UAV_Control/Rotation Angles to Direction Cosine Matrix body to earth Rotation Order: ZXY ==
  R1,R2,R3 : Inport  PortDimensions=3
  Fcn11 : Fcn  Expr=-u(1)*u(2)*u(3) + u(6)*u(4)
  Fcn12 : Fcn  Expr=-u(4)*u(3)
  Fcn13 : Fcn  Expr=u(1)*u(5)*u(3) + u(2)*u(6)
  Fcn21 : Fcn  Expr=u(1)*u(2)*u(6) + u(3)*u(4)
  Fcn22 : Fcn  Expr=u(4)*u(6)
  Fcn23 : Fcn  Expr=-u(1)*u(5)*u(6) + u(2)*u(3)
  Fcn31 : Fcn  Expr=-u(2)*u(4)
  Fcn32 : Fcn  Expr=u(1)
  Fcn33 : Fcn  Expr=u(4)*u(5)
  Mux : Mux  Inputs=2
  Subsystem : Subsystem
  sincos : Trigonometry  Operator=sincos
  DCM : Outport  PortDimensions=[3,3]
  wires:
  Fcn33/1 -> Subsystem/9(In9)
  Fcn32/1 -> Subsystem/8(In8)
  Fcn23/1 -> Subsystem/6(In6)
  Fcn22/1 -> Subsystem/5(In5)
  Fcn31/1 -> Subsystem/7(In7)
  Fcn21/1 -> Subsystem/4(In4)
  Fcn13/1 -> Subsystem/3(In3)
  Fcn12/1 -> Subsystem/2(In2)
  Fcn11/1 -> Subsystem/1(In1)
  Mux/1 -> Fcn32/1, Fcn33/1, Fcn31/1, Fcn23/1, Fcn12/1, Fcn11/1, Fcn13/1, Fcn21/1, Fcn22/1
  sincos/2 -> Mux/2
  sincos/1 -> Mux/1
  Subsystem/1(Out1) -> DCM/1
  R1,R2,R3/1 -> sincos/1

== system UAV_Control/Skew Simmetric matrix ==
  A : Inport
  Constant : Constant  Value=0
  Demux : Demux  Outputs=3
  Gain : Gain  Gain=-1
  Gain1 : Gain  Gain=-1
  Gain2 : Gain  Gain=-1
  Matrix Concatenate : Concatenate  NumInputs=3  Mode=Multidimensional array  ConcatenateDimension=2
  Mux : Mux  Inputs=3
  Mux1 : Mux  Inputs=3
  Mux2 : Mux  Inputs=3
  Reshape : Reshape  OutputDimensionality=Column vector (2-D)
  Reshape1 : Reshape  OutputDimensionality=Column vector (2-D)
  Reshape2 : Reshape  OutputDimensionality=Column vector (2-D)
  A_x : Outport
  wires:
  Gain2/1 -> Mux2/2
  Gain1/1 -> Mux1/1
  Gain/1 -> Mux/3
  Mux/1 -> Reshape/1
  Mux2/1 -> Reshape2/1
  Matrix Concatenate/1 -> A_x/1
  Reshape2/1 -> Matrix Concatenate/3
  Reshape/1 -> Matrix Concatenate/1
  Mux1/1 -> Reshape1/1
  Reshape1/1 -> Matrix Concatenate/2
  Demux/3 -> Gain1/1, Mux/2
  Constant/1 -> Mux2/3, Mux1/2, Mux/1
  Demux/1 -> Gain2/1, Mux1/3
  Demux/2 -> Gain/1, Mux2/1
  A/1 -> Demux/1

== system UAV_Control/four points moving average ==
  u : Inport
  Add : Sum  Inputs=++++
  Gain : Gain  Gain=1/4
  Gain1 : Gain  Gain=1.75
  Gain2 : Gain
  Gain3 : Gain  Gain=0.75
  Gain4 : Gain  Gain=0.5
  Memory : Memory
  Memory1 : Memory
  Memory2 : Memory
  y : Outport
  wires:
  u/1 -> Memory/1, Gain1/1
  Gain4/1 -> Add/4
  Gain2/1 -> Add/2
  Add/1 -> Gain/1
  Gain1/1 -> Add/1
  Memory2/1 -> Gain4/1
  Gain3/1 -> Add/3
  Gain/1 -> y/1
  Memory1/1 -> Memory2/1, Gain3/1
  Memory/1 -> Memory1/1, Gain2/1

== system UAV_Control/gyro ==
  In1 : Inport
  Add : Sum
  Add1 : Sum
  Band-Limited White Noise : simulink/Sources/Band-Limited White Noise  Cov=(0.03)^2  Ts=1/500  seed=[23341]
  Bias : Constant  Value=0
  Filter : TransferFcn  Numerator=[omega2^2]  Denominator=[1 2*zeta2*omega2 omega2^2]
  Gain : Gain
  Saturation : Saturate  UpperLimit=2*15  LowerLimit=-2*15
  Transfer Fcn : TransferFcn  Numerator=[omega1^2]  Denominator=[1 2*zeta1*omega1 omega1^2]
  Out1 : Outport
  wires:
  Add/1 -> Add1/1
  Saturation/1 -> Out1/1
  Bias/1 -> Add/2
  In1/1 -> Transfer Fcn/1
  Gain/1 -> Filter/1
  Filter/1 -> Saturation/1
  Band-Limited White Noise/1 -> Add1/2
  Transfer Fcn/1 -> Add/1
  Add1/1 -> Gain/1

== system UAV_Control/motor and proppeler model ==
  u : Inport
  1-D Lookup Table : Lookup_n-D  NumberOfTableDimensions=1  BreakpointsForDimension1=RPM_per  Table=Thrust_per  InternalRulePriority=Speed  RndMeth=Simplest  InputSameDT=on
  Math Function4 : Math  Operator=magnitude^2  SaturateOnIntegerOverflow=on
  Switch : Switch  Criteria=u2 > Threshold  Threshold=0.5
  correction mode : Constant  Value=c
  rotor : TransferFcn  Numerator=1  Denominator=[Tm 1]
  y : Outport
  wires:
  rotor/1 -> 1-D Lookup Table/1, Math Function4/1
  Switch/1 -> y/1
  correction mode/1 -> Switch/2
  1-D Lookup Table/1 -> Switch/1
  u/1 -> rotor/1
  Math Function4/1 -> Switch/3

== system UAV_Control/norm(u) ==
  u : Inport
  Dot Product : DotProduct  InputSameDT=on  OutDataTypeStr=Inherit: Inherit via internal rule
  Sqrt : Sqrt  SaturateOnIntegerOverflow=on
  y : Outport
  wires:
  Dot Product/1 -> Sqrt/1
  u/1 -> Dot Product/2, Dot Product/1
  Sqrt/1 -> y/1

== system UAV_Control/proppellers Resulting force and moments ==
  omega2 : Inport
  Fz : Fcn  Expr=K*(u(1)+u(2)+u(3)+u(4))
  Tx : Fcn  Expr=L*K*(u(3)-u(4))
  Ty : Fcn  Expr=L*K*(u(1)-u(2))
  Tz : Fcn  Expr=Ky*(u(1)+u(2)-u(3)-u(4))
  "Fz " : Outport
  "Tx " : Outport  Port=2
  "Ty " : Outport  Port=3
  "Tz " : Outport  Port=4
  wires:
  omega2/1 -> Ty/1, Tz/1, Tx/1, Fz/1
  Tz/1 -> "Tz "/1
  Ty/1 -> "Ty "/1
  Tx/1 -> "Tx "/1
  Fz/1 -> "Fz "/1

== system UAV_Control/sensor ==
  u : Inport
  Add1 : Sum
  Band-Limited White Noise : simulink/Sources/Band-Limited White Noise  Cov=(0.03)^2  Ts=h  seed=[23341]
  Filter : TransferFcn  Numerator=[12^2]  Denominator=[1 2*1*12 12^2]
  delay : Subsystem
  y : Outport
  wires:
  delay/1(y) -> Add1/1
  Add1/1 -> Filter/1
  Band-Limited White Noise/1 -> Add1/2
  u/1 -> delay/1(u)
  Filter/1 -> y/1

== system UAV_Control/3x3 Cross Product/Subsystem ==
  A : Inport
  B : Inport  Port=2
  Demux : Demux  Outputs=3
  Demux1 : Demux  Outputs=3
  Mux : Mux  Inputs=3
  i x j : Product  SaturateOnIntegerOverflow=on  InputSameDT=on  OutDataTypeStr=Inherit: Same as first input
  j x k : Product  SaturateOnIntegerOverflow=on  InputSameDT=on  OutDataTypeStr=Inherit: Same as first input
  k x i : Product  SaturateOnIntegerOverflow=on  InputSameDT=on  OutDataTypeStr=Inherit: Same as first input
  Out1 : Outport
  wires:
  Demux1/3 -> j x k/2
  Demux/2 -> j x k/1
  A/1 -> Demux/1
  j x k/1 -> Mux/1
  Mux/1 -> Out1/1
  Demux/3 -> k x i/1
  k x i/1 -> Mux/2
  Demux/1 -> i x j/1
  Demux1/1 -> k x i/2
  B/1 -> Demux1/1
  Demux1/2 -> i x j/2
  i x j/1 -> Mux/3

== system UAV_Control/3x3 Cross Product/Subsystem1 ==
  A : Inport
  B : Inport  Port=2
  Demux : Demux  Outputs=3
  Demux1 : Demux  Outputs=3
  Mux : Mux  Inputs=3
  i x k : Product  SaturateOnIntegerOverflow=on  InputSameDT=on  OutDataTypeStr=Inherit: Same as first input
  j x i : Product  SaturateOnIntegerOverflow=on  InputSameDT=on  OutDataTypeStr=Inherit: Same as first input
  k x j : Product  SaturateOnIntegerOverflow=on  InputSameDT=on  OutDataTypeStr=Inherit: Same as first input
  Out1 : Outport
  wires:
  j x i/1 -> Mux/3
  i x k/1 -> Mux/2
  k x j/1 -> Mux/1
  Mux/1 -> Out1/1
  Demux1/1 -> j x i/2
  Demux/2 -> j x i/1
  Demux1/3 -> i x k/2
  Demux/1 -> i x k/1
  Demux1/2 -> k x j/2
  Demux/3 -> k x j/1
  B/1 -> Demux1/1
  A/1 -> Demux/1

== system UAV_Control/ARC block/h^2 ==
  e : Inport
  phi : Inport  Port=2
  Add : Sum
  Constant3 : Constant  Value=theta_max-theta_min
  Constant6 : Constant  Value=delta
  Gain : Gain  Gain=1/(4*epsilon)
  Math Function : Math  Operator=magnitude^2  SaturateOnIntegerOverflow=on
  Math Function1 : Math  Operator=magnitude^2  SaturateOnIntegerOverflow=on
  Math Function3 : Math  Operator=magnitude^2  SaturateOnIntegerOverflow=on
  Math Function5 : Math  Operator=transpose  SaturateOnIntegerOverflow=on
  Product : Product  Multiplication=Matrix(*)
  Product1 : Product
  "alpha_s2 " : Outport
  wires:
  Constant3/1 -> Math Function/1
  e/1 -> Gain/1
  Product1/1 -> "alpha_s2 "/1
  Constant6/1 -> Math Function3/1
  Product/1 -> Add/1
  Math Function3/1 -> Add/2
  Add/1 -> Product1/1
  Math Function/1 -> Product/2
  Math Function1/1 -> Math Function5/1
  Math Function5/1 -> Product/1
  Gain/1 -> Product1/2
  phi/1 -> Math Function1/1

== system UAV_Control/DCM (body to earth) to Rotation Angles Rotation Order: ZXY/AxisRotDefault  ==
  In1 : Inport
  Action Port : ActionPort
  Fcn1 : Fcn  Expr=atan2(u[1],u[2])
  Fcn2 : Fcn  Expr=asin(u[3])
  Fcn3 : Fcn  Expr=atan2(u[4],u[5])
  Vector Concatenate : Concatenate  NumInputs=3
  Out1 : Outport
  wires:
  Fcn2/1 -> Vector Concatenate/2  "r2"
  In1/1 -> Fcn3/1, Fcn1/1, Fcn2/1
  Vector Concatenate/1 -> Out1/1
  Fcn3/1 -> Vector Concatenate/3  "r3"
  Fcn1/1 -> Vector Concatenate/1  "r1"

== system UAV_Control/DCM (body to earth) to Rotation Angles Rotation Order: ZXY/AxisRotZeroR3  ==
  In1 : Inport
  Action Port : ActionPort
  Fcn1 : Fcn  Expr=atan2(u[6],u[7])
  Fcn2 : Fcn  Expr=asin(u[3])
  Fcn3 : Fcn  Expr=0
  Vector Concatenate : Concatenate  NumInputs=3
  Out1 : Outport
  wires:
  Vector Concatenate/1 -> Out1/1
  Fcn2/1 -> Vector Concatenate/2  "r2"
  Fcn3/1 -> Vector Concatenate/3  "r3"
  In1/1 -> Fcn2/1, Fcn1/1, Fcn3/1
  Fcn1/1 -> Vector Concatenate/1  "r1"

== system UAV_Control/DCM (body to earth) to Rotation Angles Rotation Order: ZXY/Get DCM Values  ==
  In1 : Inport
  Gain1 : Gain  Gain=[1 1 -1]
  Gain2 : Gain  Gain=[1 1]
  Gain3 : Gain  Gain=[-1 1]
  Reshape : Reshape
  Reshape1 : Reshape
  Reshape2 : Reshape
  Selector1 : Selector  NumberOfDimensions=2  InputPortWidth=3  IndexOptions=Index vector (dialog),Index vector (dialog)  Indices=1,[2 1 3]  OutputSizes=1,1
  Selector2 : Selector  NumberOfDimensions=2  InputPortWidth=3  IndexOptions=Index vector (dialog),Index vector (dialog)  Indices=[2 3],3  OutputSizes=1,1
  Selector3 : Selector  NumberOfDimensions=2  InputPortWidth=3  IndexOptions=Index vector (dialog),Index vector (dialog)  Indices=2,[1 2]  OutputSizes=1,1
  Vector Concatenate : Concatenate  NumInputs=3
  Out1 : Outport
  wires:
  Selector2/1 -> Reshape1/1
  Selector1/1 -> Reshape/1
  Reshape1/1 -> Gain2/1
  Reshape2/1 -> Gain3/1
  Reshape/1 -> Gain1/1
  Selector3/1 -> Reshape2/1
  In1/1 -> Selector1/1, Selector2/1, Selector3/1
  Gain2/1 -> Vector Concatenate/2
  Gain1/1 -> Vector Concatenate/1
  Vector Concatenate/1 -> Out1/1
  Gain3/1 -> Vector Concatenate/3

== system UAV_Control/IARC, Physical Model Based Parameter Estimation (69)/Discontinuous_Proj_(49) ==
  Theta_dot : Inport
  Adapt : Inport  Port=2
  Integrator2 : Integrator  InitialCondition=theta_0  LimitOutput=on  UpperSaturationLimit=theta_max  LowerSaturationLimit=theta_min
  Product : Product
  Saturation : Saturate  UpperLimit=Theta_dot_M  LowerLimit=-Theta_dot_M
  theta dot : Scope
  Theta : Outport
  wires:
  Saturation/1 -> Integrator2/1, theta dot/1
  Product/1 -> Saturation/1
  Integrator2/1 -> Theta/1
  Adapt/1 -> Product/2
  Theta_dot/1 -> Product/1

== system UAV_Control/IARC, Physical Model Based Parameter Estimation (69)/Epsilon ==
  y_f : Inport
  Phi_f : Inport  Port=2
  Theta_hat : Inport  Port=3
  Product1 : Product
  Subtract : Sum  Inputs=+-
  Epsilon : Outport
  wires:
  Theta_hat/1 -> Product1/2
  Phi_f/1 -> Product1/1
  Product1/1 -> Subtract/2  "Yp_hat"
  Subtract/1 -> Epsilon/1
  y_f/1 -> Subtract/1  "Yp"

== system UAV_Control/IARC, Physical Model Based Parameter Estimation (69)/Filter ==
  y : Inport
  "Phi " : Inport  Port=2
  Mux1 : Mux  Inputs=2
  Mux2 : Mux  Inputs=2
  filter : TransferFcn  Denominator=[Tau 1]
  "filter " : TransferFcn  Denominator=[Tau 1]
  gamma : Scope
  gamma1 : Scope
  y_f : Outport
  Phi_f : Outport  Port=2
  wires:
  Mux2/1 -> gamma1/1
  "Phi "/1 -> filter/1, Mux2/1
  Mux1/1 -> gamma/1
  y/1 -> "filter "/1, Mux1/1
  "filter "/1 -> Mux1/2, y_f/1
  filter/1 -> Phi_f/1, Mux2/2

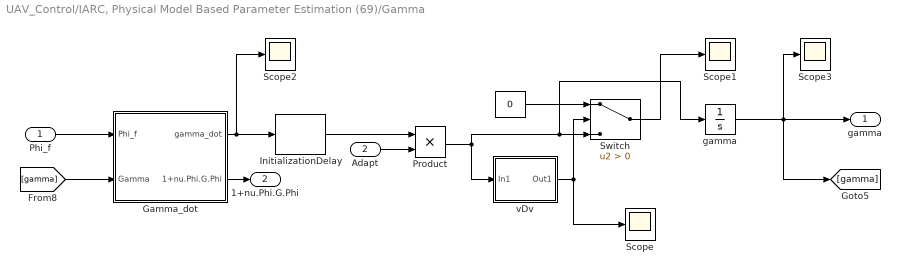
== system UAV_Control/IARC, Physical Model Based Parameter Estimation (69)/Gamma ==
  Phi_f : Inport
  Adapt : Inport  Port=2
  " " : Constant  Value=0
  Gamma_dot : Subsystem
  InitializationDelay : $bdroot/InitializationDelay  t0=t1
  Product : Product
  Scope{,1..3} (4 alike) : Scope
  Switch : Switch  Criteria=u2 > Threshold
  "gamma " : Integrator  InitialCondition=gamma0  LimitOutput=on  UpperSaturationLimit=Rho_M  LowerSaturationLimit=Rho_L
  vDv : Subsystem
  " gamma" : Outport
  " 1+nu.Phi.G.Phi" : Outport  Port=2
  wires:
  Switch/1 -> Scope1/1
  Product/1 -> Switch/3, "gamma "/1, vDv/1(In1)
  Gamma_dot/2(" 1+nu.Phi.G.Phi") -> " 1+nu.Phi.G.Phi"/1
  [gamma] -> Gamma_dot/2(Gamma)
  Gamma_dot/1(gamma_dot) -> InitializationDelay/1, Scope2/1
  Phi_f/1 -> Gamma_dot/1(Phi_f)
  vDv/1(Out1) -> Switch/2, Scope/1
  " "/1 -> Switch/1
  "gamma "/1 -> " gamma"/1, [gamma], Scope3/1
  Adapt/1 -> Product/2
  InitializationDelay/1 -> Product/1

== system UAV_Control/Rigid Body Force Equations/On ground Reaction acceleration adjustment ==
  X : Inport
  ab_in : Inport  Port=2
  a_thrust : Inport  Port=3
  Compare To Zero : simulink/Logic and Bit Operations/Compare To Zero  relop=<=  OutDataTypeStr=boolean
  Logical Operator : Logic  AllPortsSameDT=off  OutDataTypeStr=boolean
  On Ground Condition : simulink/Logic and Bit Operations/Compare To Constant  relop=<=  const=Zg  OutDataTypeStr=boolean
  Product3 : Product
  Selector1 : Selector  InputPortWidth=3  IndexOptions=Index vector (dialog)  Indices=[3]  OutputSizes=1
  deliver thrust : Logic  Operator=NOT  AllPortsSameDT=off  OutDataTypeStr=boolean
  ab_out : Outport
  wires:
  Logical Operator/1 -> deliver thrust/1
  Selector1/1 -> On Ground Condition/1
  X/1 -> Selector1/1
  Product3/1 -> ab_out/1
  On Ground Condition/1 -> Logical Operator/1
  Compare To Zero/1 -> Logical Operator/2
  a_thrust/1 -> Compare To Zero/1
  ab_in/1 -> Product3/2
  deliver thrust/1 -> Product3/1

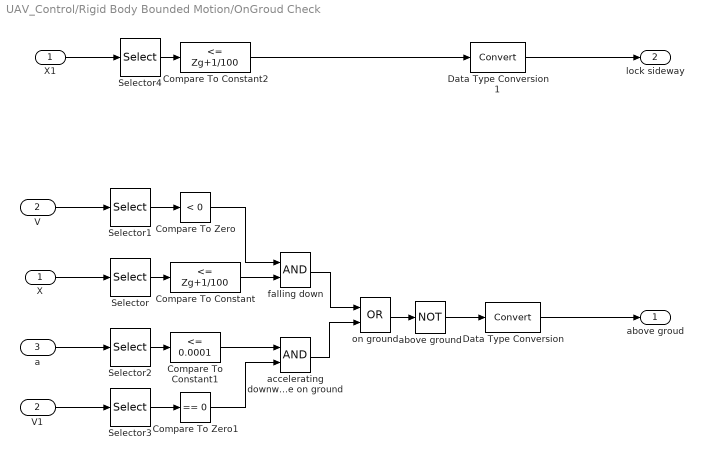
== system UAV_Control/Rigid Body Bounded Motion/OnGroud Check ==
  X : Inport
  V : Inport  Port=2
  a : Inport  Port=3
  Compare To Constant : simulink/Logic and Bit Operations/Compare To Constant  relop=<=  const=Zg+1/100  OutDataTypeStr=boolean
  Compare To Constant1 : simulink/Logic and Bit Operations/Compare To Constant  relop=<=  const=0.0001  OutDataTypeStr=boolean
  Compare To Constant2 : simulink/Logic and Bit Operations/Compare To Constant  relop=<=  const=Zg+1/100  OutDataTypeStr=boolean
  Compare To Zero : simulink/Logic and Bit Operations/Compare To Zero  relop=<  OutDataTypeStr=boolean
  Compare To Zero1 : simulink/Logic and Bit Operations/Compare To Zero  relop===  OutDataTypeStr=boolean
  Data Type Conversion : DataTypeConversion
  Data Type Conversion1 : DataTypeConversion
  Selector{,1..4} (5 alike) : Selector  InputPortWidth=3  IndexOptions=Index vector (dialog)  Indices=[3]  OutputSizes=1
  V1 : InportShadow  Port=2
  X1 : InportShadow
  above ground : Logic  Operator=NOT  AllPortsSameDT=off  OutDataTypeStr=boolean
  accelerating downward while on ground : Logic  AllPortsSameDT=off  OutDataTypeStr=boolean
  falling down : Logic  AllPortsSameDT=off  OutDataTypeStr=boolean
  on ground : Logic  Operator=OR  AllPortsSameDT=off  OutDataTypeStr=boolean
  above groud : Outport
  lock sideway : Outport  Port=2
  wires:
  Data Type Conversion/1 -> above groud/1
  accelerating downward while on ground/1 -> on ground/2
  Compare To Zero1/1 -> accelerating downward while on ground/2
  Compare To Constant1/1 -> accelerating downward while on ground/1
  falling down/1 -> on ground/1
  Selector3/1 -> Compare To Zero1/1
  V1/1 -> Selector3/1
  Compare To Constant/1 -> falling down/2
  Compare To Zero/1 -> falling down/1
  Selector2/1 -> Compare To Constant1/1
  a/1 -> Selector2/1
  above ground/1 -> Data Type Conversion/1
  V/1 -> Selector1/1
  X/1 -> Selector/1
  on ground/1 -> above ground/1
  Selector/1 -> Compare To Constant/1
  Selector1/1 -> Compare To Zero/1
  Selector4/1 -> Compare To Constant2/1
  X1/1 -> Selector4/1
  Compare To Constant2/1 -> Data Type Conversion1/1
  Data Type Conversion1/1 -> lock sideway/1
